simulink model "untitled1"  (R2022b)
settings: Solver=VariableStepAuto  StartTime=0.0  StopTime=10.0  RelTol=1e-3

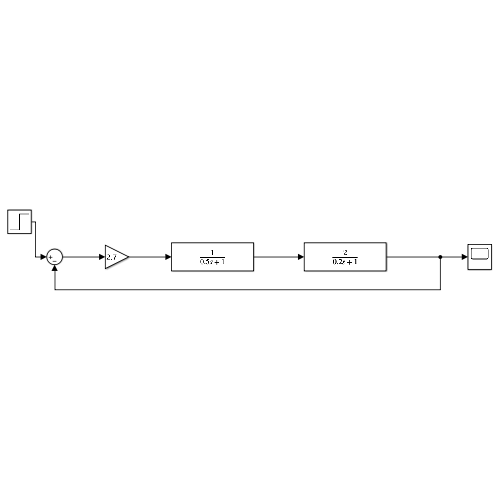
[thumbnail: Simulink's stored preview of the top-level diagram]
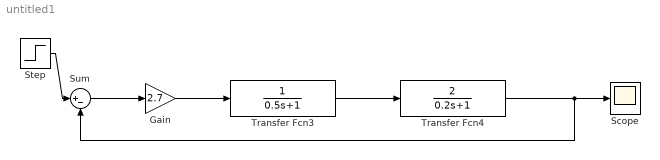
== system untitled1 ==
  Gain : Gain  Gain=2.7
  Scope : Scope
  Step : Step  SampleTime=0
  Sum : Sum  Inputs=|+-
  Transfer Fcn3 : TransferFcn  Denominator=[0.5 1]
  Transfer Fcn4 : TransferFcn  Numerator=[2]  Denominator=[0.2 1]
  wires:
  Step/1 -> Sum/1
  Sum/1 -> Gain/1
  Gain/1 -> Transfer Fcn3/1
  Transfer Fcn3/1 -> Transfer Fcn4/1
  Transfer Fcn4/1 -> Sum/2, Scope/1
